simulink model "RB_KAIROS_impControl_repulsive"  (R2020b)
(part 8 of 17)

t16463 = t5538+t5554+t5559+t5562+t6273+t6622+t7789+t8207+t8776+t8806+t9051+t9058+t9390+t9445+t10331+t10348+t10391+t10526+t10527+t10572+t10582+t10671+t10903+t10914+t10916+t11226+t11229+t11392+t11402+t11526+t11527+t11537+t11557+t11731+t11732+t11747+t11777+t12054+t12076+t12297+t12302+t12310+t12561+t12837+t13086+t13093+t13246+t13261+t13309+t13696+t13936+t13949+t14074+t14103+t14110+t14129+t14146+t14237+t14357+t14359+t14389+t14552+t14778+t14788+t15029+t15035+t15264+t15266+t15402+t15419+t15421+t15441+t15443+t15504+t15505+t15513+t15527+t15612+t15956+t15961+t15991+t15993+t15999+t16000+t16019+t16021;
t16464 = t5516+t5522+t5589+t5597+t6258+t6613+t7763+t8161+t8861+t8902+t9085+t9088+t9406+t9476+t10324+t10356+t10401+t10512+t10538+t10559+t10594+t10651+t10900+t10919+t10934+t11246+t11267+t11359+t11365+t11539+t11540+t11566+t11601+t11706+t11713+t11715+t11800+t12043+t12084+t12309+t12313+t12336+t12555+t12845+t13104+t13112+t13270+t13282+t13316+t13708+t13918+t13933+t14059+t14102+t14109+t14118+t14133+t14236+t14356+t14358+t14378+t14551+t14811+t14829+t15051+t15060+t15246+t15261+t15399+t15423+t15425+t15433+t15438+t15509+t15510+t15514+t15524+t15613+t15947+t15954+t15988+t15990+t16002+t16003+t16022+t16024;
t16465 = t5514+t5527+t5571+t5575+t6258+t6613+t7777+t8172+t8844+t8878+t9078+t9084+t9425+t9485+t10324+t10356+t10401+t10512+t10538+t10559+t10594+t10651+t10900+t10919+t10934+t11254+t11258+t11359+t11365+t11539+t11540+t11578+t11596+t11706+t11713+t11715+t11812+t12043+t12084+t12309+t12313+t12340+t12555+t12845+t13109+t13116+t13277+t13286+t13318+t13710+t13918+t13933+t14059+t14102+t14109+t14118+t14133+t14236+t14356+t14358+t14378+t14551+t14817+t14826+t15052+t15058+t15246+t15261+t15399+t15423+t15425+t15433+t15438+t15509+t15510+t15514+t15524+t15613+t15947+t15954+t15988+t15990+t16002+t16003+t16022+t16024;
t16466 = xd.*(-t5516-t5522-t5589-t5597-t6249-t6602-t7763-t8161+t8844+t8878+t9078+t9084+t9425+t9485+t10324+t10356+t10401+t10512+t10538+t10559+t10594+t10651+t10900+t10919+t10934+t11254+t11258+t11359+t11365+t11539+t11540+t11578+t11596+t11706+t11713+t11715+t11812+t12043+t12084+t12309+t12313+t12340+t12555+t12845+t13109+t13116+t13277+t13286+t13318+t13710+t13918+t13933+t14059+t14102+t14109+t14118+t14133+t14236+t14356+t14358+t14378+t14551+t14817+t14826+t15052+t15058+t15246+t15261+t15399+t15423+t15425+t15433+t15438+t15509+t15510+t15514+t15524+t15613+t15947+t15954+t15988+t15990+t16002+t16003+t16022+t16024);
t16467 = t5262+t5587+t6225+t6309+t6356+t6586+t7355+t7374+t7805+t7807+t7894+t8231+t8232+t8294+t8836+t8841+t9398+t9420+t9515+t9523+t9569+t9585+t9608+t9666+t9791+t9838+t9862+t9897+t10151+t10162+t10252+t10712+t10957+t11084+t11615+t11628+t11748+t11765+t11773+t11774+t12066+t12098+t12177+t12194+t12228+t12261+t12274+t12305+t12316+t12736+t12737+t12836+t13544+t13557+t13707+t13714+t13815+t13871+t13875+t13916+t13927+t13942+t14028+t14067+t14084+t14157+t14164+t14179+t14253+t14314+t15094+t15104+t15137+t15145+t15230+t15231+t15296+t15299+t15302+t15305+t15311+t15409+t15414+t15422+t15485+t15530+t15895+t15896+t15915+t15916+t15936+t15937+t15974+t15975;
t16469 = t5252+t5569+t6239+t6309+t6356+t6597+t7332+t7387+t7792+t7821+t7876+t8231+t8232+t8282+t8836+t8841+t9419+t9441+t9515+t9523+t9569+t9585+t9608+t9666+t9791+t9838+t9874+t9901+t10151+t10162+t10242+t10712+t10957+t11080+t11615+t11628+t11758+t11773+t11774+t11775+t12071+t12098+t12177+t12194+t12228+t12265+t12277+t12305+t12316+t12737+t12739+t12836+t13546+t13554+t13707+t13714+t13819+t13871+t13875+t13919+t13923+t13942+t14028+t14067+t14084+t14157+t14164+t14181+t14253+t14314+t15096+t15100+t15137+t15145+t15230+t15231+t15299+t15301+t15302+t15303+t15311+t15409+t15414+t15422+t15485+t15530+t15895+t15896+t15915+t15916+t15936+t15937+t15974+t15975;
t16471 = t16470.*yd;
t16480 = t3860+t3982+t4535+t4632+t5577+t5579+t6236+t6324+t6371+t6593+t7161+t7166+t7429+t7444+t7452+t7493+t7502+t7519+t7589+t7651+t7655+t7956+t8024+t8142+t8147+t8233+t8280+t8349+t8357+t8372+t8393+t8414+t8487+t8797+t8842+t9477+t9707+t9741+t10070+t10071+t10074+t10084+t10085+t10089+t10316+t10344+t10455+t10557+t10585+t10649+t10904+t10917+t11255+t11721+t11791+t11793+t11794+t11802+t11805+t11806+t12134+t12164+t12315+t12323+t12430+t12631+t12657+t12693+t12697+t12712+t13065+t13268+t13783+t13784+t13790+t13808+t13809+t13810+t13811+t13812+t14043+t14056+t14062+t14317+t14321+t14367+t14435+t14590+t14601+t14750+t15247+t15248+t15249+t15250+t15262+t15263+t15330+t15331+t15466+t15467+t15567+t15573+t15624+t15629+t15633+t15735+t15934+t15935+t15938+t15939+t16043+t16046+t16060+t16064;
t16483 = t16482.*xd;
t16484 = t3904+t3989+t4538+t4667+t5639+t5641+t6274+t6294+t6358+t6621+t7131+t7137+t7418+t7443+t7468+t7477+t7503+t7531+t7590+t7681+t7683+t7943+t8039+t8169+t8171+t8262+t8281+t8351+t8370+t8380+t8399+t8407+t8471+t8784+t8879+t9448+t9759+t9770+t10063+t10064+t10098+t10100+t10103+t10104+t10360+t10362+t10471+t10556+t10584+t10648+t10899+t10925+t11272+t11712+t11750+t11751+t11778+t11779+t11780+t11781+t12161+t12189+t12345+t12351+t12447+t12635+t12686+t12717+t12722+t12729+t13080+t13271+t13759+t13760+t13778+t13779+t13781+t13782+t13821+t13838+t14066+t14086+t14090+t14320+t14338+t14384+t14443+t14602+t14617+t14755+t15232+t15233+t15234+t15235+t15244+t15245+t15359+t15362+t15474+t15475+t15577+t15582+t15631+t15638+t15640+t15738+t15923+t15924+t15925+t15926+t16047+t16050+t16065+t16068;
t16188 = t16187.*yd;
t16205 = t16204.*yd;
t16276 = t16275.*yd;
t16292 = t16291.*yd;
t16336 = t16335.*yd;
t16368 = t16367.*xd;
t16412 = t16411.*yd;
t16420 = t16419.*xd;
t16454 = t16453.*yd;
t16468 = t16467.*xd;
